simulink model "sistem_full"  (R2020b)
settings: Solver=ode45  StartTime=0.0  StopTime=10.0  MaxStep=0.01  RelTol=1e-3
undefined symbols (not defined in the file or in its folder): K_d, K_p, params, r_des
(part 2 of 2)

== matlab function sistem_full/MATLAB Function19 ==
  data: t input; coeff output; r_0 input; r_end input
function coeff  = calculation_coefficients(t, r_0, r_end)

x_0 = r_0;
x_dot_0 = 0;
x_ddot_0 = 0;

x_des = r_end;
x_dot_des = 0;
x_ddot_des = 0;

waypoints = [x_0    x_dot_0     x_ddot_0;
             x_des  x_dot_des   x_ddot_des]';
t = [0 t];

time_size = size(t);
n = 0;
%T = linspace(0, time_size(2) - 1, point(2));


border_conditions_sigm = reshape(waypoints(:, n + 1 : n + 2),1,[]);
%disp(border_conditions_sigm)

coeff = zeros(6, 1);

parameters = [1 * (t(n + 1) ^ 5), 1 * (t(n + 1) ^ 4), 1 * (t(n + 1) ^ 3), 1 * (t(n + 1) ^ 2), 1 * (t(n + 1) ^ 1), 1 * (t(n + 1) ^ 0);
              5 * (t(n + 1) ^ 4), 4 * (t(n + 1) ^ 3), 3 * (t(n + 1) ^ 2), 2 * (t(n + 1) ^ 1), 1 * (t(n + 1) ^ 0), 0 * (t(n + 1) ^ 0);
              20 * (t(n + 1) ^ 3), 12 * (t(n + 1) ^ 2), 6 * (t(n + 1) ^ 1), 2 * (t(n + 1) ^ 0), 0 * (t(n + 1) ^ 0), 0 * (t(n + 1) ^ 0);
              1 * (t(n + 2) ^ 5), 1 * (t(n + 2) ^ 4), 1 * (t(n + 2) ^ 3), 1 * (t(n + 2) ^ 2), 1 * (t(n + 2) ^ 1), 1 * (t(n + 2) ^ 0);
              5 * (t(n + 2) ^ 4), 4 * (t(n + 2) ^ 3), 3 * (t(n + 2) ^ 2), 2 * (t(n + 2) ^ 1), 1 * (t(n + 2) ^ 0), 0 * (t(n + 2) ^ 0);
              20 * (t(n + 2) ^ 3), 12 * (t(n + 2) ^ 2), 6 * (t(n + 2) ^ 1), 2 * (t(n + 2) ^ 0), 0 * (t(n + 2) ^ 0), 0 * (t(n + 2) ^ 0)];

coeff = inv(parameters) * border_conditions_sigm';

== matlab function sistem_full/MATLAB Function20 ==
  data: coeff input; pos output; clock input; vel output; acc output
function [pos, vel, acc] = trajectories_calculation(coeff, clock)

T_p = [clock^5      clock^4     clock^3     clock^2     clock   1]';
T_v = [5*clock^4    4*clock^3   3*clock^2   2*clock     1       0]';
T_a = [20*clock^3   12*clock^2  6*clock     2           0       0]';

pos = sum(coeff.*T_p);
vel = sum(coeff.*T_v);
acc = sum(coeff.*T_a);

== matlab function sistem_full/MATLAB Function21 ==
  data: t input; coeff output; r_0 input; r_end input
function coeff  = calculation_coefficients(t, r_0, r_end)

x_0 = r_0;
x_dot_0 = 14.1;
x_ddot_0 = 0;

x_des = r_end;
x_dot_des = 14.1;
x_ddot_des = 0;

waypoints = [x_0    x_dot_0     x_ddot_0;
             x_des  x_dot_des   x_ddot_des]';
t = [0 t];

time_size = size(t);
n = 0;
%T = linspace(0, time_size(2) - 1, point(2));


border_conditions_sigm = reshape(waypoints(:, n + 1 : n + 2),1,[]);
%disp(border_conditions_sigm)

coeff = zeros(6, 1);

parameters = [1 * (t(n + 1) ^ 5), 1 * (t(n + 1) ^ 4), 1 * (t(n + 1) ^ 3), 1 * (t(n + 1) ^ 2), 1 * (t(n + 1) ^ 1), 1 * (t(n + 1) ^ 0);
              5 * (t(n + 1) ^ 4), 4 * (t(n + 1) ^ 3), 3 * (t(n + 1) ^ 2), 2 * (t(n + 1) ^ 1), 1 * (t(n + 1) ^ 0), 0 * (t(n + 1) ^ 0);
              20 * (t(n + 1) ^ 3), 12 * (t(n + 1) ^ 2), 6 * (t(n + 1) ^ 1), 2 * (t(n + 1) ^ 0), 0 * (t(n + 1) ^ 0), 0 * (t(n + 1) ^ 0);
              1 * (t(n + 2) ^ 5), 1 * (t(n + 2) ^ 4), 1 * (t(n + 2) ^ 3), 1 * (t(n + 2) ^ 2), 1 * (t(n + 2) ^ 1), 1 * (t(n + 2) ^ 0);
              5 * (t(n + 2) ^ 4), 4 * (t(n + 2) ^ 3), 3 * (t(n + 2) ^ 2), 2 * (t(n + 2) ^ 1), 1 * (t(n + 2) ^ 0), 0 * (t(n + 2) ^ 0);
              20 * (t(n + 2) ^ 3), 12 * (t(n + 2) ^ 2), 6 * (t(n + 2) ^ 1), 2 * (t(n + 2) ^ 0), 0 * (t(n + 2) ^ 0), 0 * (t(n + 2) ^ 0)];

coeff = inv(parameters) * border_conditions_sigm';

== matlab function sistem_full/MATLAB Function22 ==
  data: r_des input; F_T output; Y output; fi_des output; x_ddot input; y_ddot input; z_ddot input; params input; mode input; theta_des output; psi_des output
function [F_T, Y, fi_des, theta_des, psi_des] = fcn(r_des, x_ddot, y_ddot, z_ddot, params, mode)

if mode == 0
    
    F_T = params.m * (z_ddot + params.g);
    Y = 0;

    fi_des = (1 / params.g) * (x_ddot * sin(r_des.psi) - y_ddot * cos(r_des.psi));
    theta_des = (1 / params.g) * (x_ddot * cos(r_des.psi) + y_ddot * sin(r_des.psi));
    psi_des = r_des.psi;
    
elseif mode == 1
    
    %F_T = params.m * x_ddot + params.k_x * x_dot;

    F_T = params.m * x_ddot + r_des.x_dot;
    Y = params.m * params.g;

    fi_des = r_des.fi;
    theta_des = (params.m / (params.k_x * r_des.x_dot)) * (y_ddot * sin(r_des.fi) - z_ddot * cos(r_des.fi));
    psi_des = (params.m / (params.k_x * r_des.x_dot)) * (y_ddot * cos(r_des.fi) + z_ddot * sin(r_des.fi));

    %theta_des = (params.m / F_T) * (y_ddot * sin(r_des.fi) - z_ddot * cos(r_des.fi));
    %psi_des = (params.m / F_T) * (y_ddot * cos(r_des.fi) + z_ddot * sin(r_des.fi));
    
else 
    
    F_T = params.m * (z_ddot + params.g);
    Y = 0;

    fi_des = (1 / params.g) * (x_ddot * sin(r_des.psi) - y_ddot * cos(r_des.psi));
    theta_des = (1 / params.g) * (x_ddot * cos(r_des.psi) + y_ddot * sin(r_des.psi));
    psi_des = r_des.psi;
    
end

== matlab function sistem_full/MATLAB Function23 ==
  data: alpha_1 output; alpha_2 output; alpha_3 output; alpha_4 output; F_T input; Y input; w output; M_x input; M_y input; M_z input; x_dot input; params input; alpha_L output; alpha_R output; alpha_H output; alpha_F output; mode input
function [alpha_1, alpha_2, alpha_3, alpha_4, w, alpha_L, alpha_R, alpha_H, alpha_F] = fcn(F_T, Y, M_x, M_y, M_z, x_dot, params, mode)

if mode == 0
    
    alpha_1 = (1 / (4 * params.k_Y)) * (F_T + M_x + M_y + M_z) - 7;
    alpha_2 = (1 / (4 * params.k_Y)) * (F_T + M_x - M_y - M_z);
    alpha_3 = (1 / (4 * params.k_Y)) * (F_T - M_x + M_y - M_z) - 7;
    alpha_4 = (1 / (4 * params.k_Y)) * (F_T - M_x - M_y + M_z);
    
    w = params.w_0;
    alpha_L = -7;
    alpha_R = -7;
    alpha_H = 0;
    alpha_F = 0;
    
elseif mode == 1
    
    alpha_1 = 7.5;
    alpha_2 = 7.5;
    alpha_3 = 7.5;
    alpha_4 = 7.5;

    w = (50000 * F_T + 245100) / 77;

    alpha_L = (500 * M_x + 500 * Y + 102201 * params.S_k * params.rho - 14630 * params.S_k * params.rho * x_dot) / (30 * params.S_k * params.rho * (70 * x_dot - 489));
    alpha_R = - (500 * M_x - 500 * Y - 102201 * params.S_k * params.rho + 14630 * params.S_k * params.rho * x_dot) / (30 * params.S_k * params.rho * (70 * x_dot - 489));
    alpha_H = (125 * M_y) / (3 * params.S_h * params.rho * (70 * x_dot - 489));
    alpha_F = (125 * M_z) / (3 * params.S_f * params.rho * (70 * x_dot - 489));
    
else
    
    alpha_1 = (1 / (4 * params.k_Y)) * (F_T + M_x + M_y + M_z) - 7;
    alpha_2 = (1 / (4 * params.k_Y)) * (F_T + M_x - M_y - M_z);
    alpha_3 = (1 / (4 * params.k_Y)) * (F_T - M_x + M_y - M_z) - 7;
    alpha_4 = (1 / (4 * params.k_Y)) * (F_T - M_x - M_y + M_z);
    
    w = params.w_0;
    alpha_L = -7;
    alpha_R = -7;
    alpha_H = 0;
    alpha_F = 0;
    
end

== matlab function sistem_full/MATLAB Function6 ==
  data: coeff input; pos output; clock input; vel output; acc output
function [pos, vel, acc] = trajectories_calculation(coeff, clock)

T_p = [clock^5      clock^4     clock^3     clock^2     clock   1]';
T_v = [5*clock^4    4*clock^3   3*clock^2   2*clock     1       0]';
T_a = [20*clock^3   12*clock^2  6*clock     2           0       0]';

pos = sum(coeff.*T_p);
vel = sum(coeff.*T_v);
acc = sum(coeff.*T_a);

== matlab function sistem_full/MATLAB Function ==
  data: coeff input; pos output; clock input; vel output; acc output
function [pos, vel, acc] = trajectories_calculation(coeff, clock)

T_p = [clock^5      clock^4     clock^3     clock^2     clock   1]';
T_v = [5*clock^4    4*clock^3   3*clock^2   2*clock     1       0]';
T_a = [20*clock^3   12*clock^2  6*clock     2           0       0]';

pos = sum(coeff.*T_p);
vel = sum(coeff.*T_v);
acc = sum(coeff.*T_a);

== matlab function sistem_full/MATLAB Function8 ==
  data: t input; coeff output; r_0 input; r_end input
function coeff  = calculation_coefficients(t, r_0, r_end)

x_0 = r_0;
x_dot_0 = 0;
x_ddot_0 = 0;

x_des = r_end;
x_dot_des = 0;
x_ddot_des = 0;

waypoints = [x_0    x_dot_0     x_ddot_0;
             x_des  x_dot_des   x_ddot_des]';
t = [0 t];

time_size = size(t);
n = 0;
%T = linspace(0, time_size(2) - 1, point(2));


border_conditions_sigm = reshape(waypoints(:, n + 1 : n + 2),1,[]);
%disp(border_conditions_sigm)

coeff = zeros(6, 1);

parameters = [1 * (t(n + 1) ^ 5), 1 * (t(n + 1) ^ 4), 1 * (t(n + 1) ^ 3), 1 * (t(n + 1) ^ 2), 1 * (t(n + 1) ^ 1), 1 * (t(n + 1) ^ 0);
              5 * (t(n + 1) ^ 4), 4 * (t(n + 1) ^ 3), 3 * (t(n + 1) ^ 2), 2 * (t(n + 1) ^ 1), 1 * (t(n + 1) ^ 0), 0 * (t(n + 1) ^ 0);
              20 * (t(n + 1) ^ 3), 12 * (t(n + 1) ^ 2), 6 * (t(n + 1) ^ 1), 2 * (t(n + 1) ^ 0), 0 * (t(n + 1) ^ 0), 0 * (t(n + 1) ^ 0);
              1 * (t(n + 2) ^ 5), 1 * (t(n + 2) ^ 4), 1 * (t(n + 2) ^ 3), 1 * (t(n + 2) ^ 2), 1 * (t(n + 2) ^ 1), 1 * (t(n + 2) ^ 0);
              5 * (t(n + 2) ^ 4), 4 * (t(n + 2) ^ 3), 3 * (t(n + 2) ^ 2), 2 * (t(n + 2) ^ 1), 1 * (t(n + 2) ^ 0), 0 * (t(n + 2) ^ 0);
              20 * (t(n + 2) ^ 3), 12 * (t(n + 2) ^ 2), 6 * (t(n + 2) ^ 1), 2 * (t(n + 2) ^ 0), 0 * (t(n + 2) ^ 0), 0 * (t(n + 2) ^ 0)];

coeff = inv(parameters) * border_conditions_sigm';

== matlab function sistem_full/Subsystem2/MATLAB Function6 ==
  data: x_des input; x_ddot output; x_dot_des input; x_ddot_des input; y_des input; y_dot_des input; y_ddot_des input; z_des input; z_dot_des input; z_ddot_des input; x input; x_dot input; y input; y_dot input; z input; z_dot input; K_p input; K_d input; y_ddot output; z_ddot output; mode input
function [x_ddot,y_ddot,z_ddot] = fcn(x_des, x_dot_des, x_ddot_des, y_des, y_dot_des, y_ddot_des, z_des, z_dot_des, z_ddot_des, ...
                                      x, x_dot, y, y_dot, z, z_dot, K_p, K_d, mode)

if mode == 0
    
    x_ddot = x_ddot_des + abs(K_d.ver.x) * (x_dot_des - x_dot) + abs(K_p.ver.x) * (x_des - x);
    y_ddot = y_ddot_des + abs(K_d.ver.y) * (y_dot_des - y_dot) + abs(K_p.ver.y) * (y_des - y);
    z_ddot = z_ddot_des + abs(K_d.ver.z) * (z_dot_des - z_dot) + abs(K_p.ver.z) * (z_des - z);

elseif mode == 1
    
    x_ddot = x_ddot_des + abs(K_d.hor.x) * (x_dot_des - x_dot) + abs(K_p.hor.x) * (x_des - x);
    y_ddot = y_ddot_des + abs(K_d.hor.y) * (y_dot_des - y_dot) + abs(K_p.hor.y) * (y_des - y);
    z_ddot = z_ddot_des + abs(K_d.hor.z) * (z_dot_des - z_dot) + abs(K_p.hor.z) * (z_des - z);
    
else
    
    x_ddot = x_ddot_des + abs(K_d.ver.x) * (x_dot_des - x_dot) + abs(K_p.ver.x) * (x_des - x);
    y_ddot = y_ddot_des + abs(K_d.ver.y) * (y_dot_des - y_dot) + abs(K_p.ver.y) * (y_des - y);
    z_ddot = z_ddot_des + abs(K_d.ver.z) * (z_dot_des - z_dot) + abs(K_p.ver.z) * (z_des - z);
    
end

== matlab function sistem_full/Subsystem3/MATLAB Function8 ==
  data: fi_des input; theta_des input; psi_des input; r_des input; fi input; fi_dot input; theta input; theta_dot input; psi input; psi_dot input; M_x output; K_p input; K_d input; params input; M_y output; M_z output; mode input
function [M_x, M_y, M_z] = fcn(fi_des, theta_des, psi_des, r_des, fi, fi_dot, theta, theta_dot, psi, psi_dot, K_p, K_d, params, mode)

if mode == 0

    M_x = (params.ver.J_xx / params.ver.L_x) * (r_des.fi_ddot + abs(K_d.ver.fi) * (r_des.fi_dot - fi_dot) + abs(K_p.ver.fi) * (fi_des - fi));
    M_y = (params.ver.J_yy / params.ver.L_y) * (r_des.theta_ddot + abs(K_d.ver.theta) * (r_des.theta_dot - theta_dot) + abs(K_p.ver.theta) * (theta_des - theta));
    M_z = (params.ver.J_zz / params.ver.L_z) * (r_des.psi_ddot + abs(K_d.ver.psi) * (r_des.psi_dot - psi_dot) + abs(K_p.ver.psi) * (psi_des - psi));
    
elseif mode == 1
    
    M_x = (params.hor.J_xx / params.hor.L_x) * (r_des.fi_ddot + abs(K_d.hor.fi) * (r_des.fi_dot - fi_dot) + abs(K_p.hor.fi) * (fi_des - fi));
    M_y = (params.hor.J_yy / params.hor.L_y) * (r_des.theta_ddot + abs(K_d.hor.theta) * (r_des.theta_dot - theta_dot) + abs(K_p.hor.theta) * (theta_des - theta));
    M_z = (params.hor.J_zz / params.hor.L_z) * (r_des.psi_ddot + abs(K_d.hor.psi) * (r_des.psi_dot - psi_dot) + abs(K_p.hor.psi) * (psi_des - psi));
    
else 
    
    M_x = (params.ver.J_xx / params.ver.L_x) * (r_des.fi_ddot + abs(K_d.ver.fi) * (r_des.fi_dot - fi_dot) + abs(K_p.ver.fi) * (fi_des - fi));
    M_y = (params.ver.J_yy / params.ver.L_y) * (r_des.theta_ddot + abs(K_d.ver.theta) * (r_des.theta_dot - theta_dot) + abs(K_p.ver.theta) * (theta_des - theta));
    M_z = (params.ver.J_zz / params.ver.L_z) * (r_des.psi_ddot + abs(K_d.ver.psi) * (r_des.psi_dot - psi_dot) + abs(K_p.ver.psi) * (psi_des - psi));
    
end

== matlab function sistem_full/MATLAB Function24 ==
  data: F_x input; x_ddot output; F_y input; F_z input; Y input; x_dot input; params input; y_ddot output; z_ddot output
function [x_ddot, y_ddot, z_ddot] = fcn(F_x, F_y, F_z, Y, x_dot, params)

x_ddot = (1 / params.m) * (F_x - params.k_x * x_dot);

%x_ddot = (1 / params.m) * (F_x);
y_ddot = (1 / params.m) * F_y;
z_ddot = (1 / params.m) * (F_z + Y - params.m * params.g);

== stateflow chart sistem_full/Chart2 ==
  state Vertical_flight
    mode = 0
    sigma = 0
  state Horizontal_flight
    mode = 1
    sigma = 90
  (default) -> Vertical_flight
  Horizontal_flight -> Vertical_flight : [x_dot_des < 14.1]
  Vertical_flight -> Horizontal_flight : [x_dot_des > 14.1]
  data: mode output; x_dot_des input; sigma output

== matlab function sistem_full/MATLAB Function25 ==
  data: coeff input; pos output; clock input; vel output; acc output
function [pos, vel, acc] = trajectories_calculation(coeff, clock)

T_p = [clock^5      clock^4     clock^3     clock^2     clock   1]';
T_v = [5*clock^4    4*clock^3   3*clock^2   2*clock     1       0]';
T_a = [20*clock^3   12*clock^2  6*clock     2           0       0]';

pos = sum(coeff.*T_p);
vel = sum(coeff.*T_v);
acc = sum(coeff.*T_a);

== matlab function sistem_full/MATLAB Function26 ==
  data: t input; coeff output; r_0 input; r_end input
function coeff  = calculation_coefficients(t, r_0, r_end)

x_0 = r_0;
x_dot_0 = 0;
x_ddot_0 = 0;

x_des = r_end;
x_dot_des = 0;
x_ddot_des = 0;

waypoints = [x_0    x_dot_0     x_ddot_0;
             x_des  x_dot_des   x_ddot_des]';
t = [0 t];

time_size = size(t);
n = 0;
%T = linspace(0, time_size(2) - 1, point(2));


border_conditions_sigm = reshape(waypoints(:, n + 1 : n + 2),1,[]);
%disp(border_conditions_sigm)

coeff = zeros(6, 1);

parameters = [1 * (t(n + 1) ^ 5), 1 * (t(n + 1) ^ 4), 1 * (t(n + 1) ^ 3), 1 * (t(n + 1) ^ 2), 1 * (t(n + 1) ^ 1), 1 * (t(n + 1) ^ 0);
              5 * (t(n + 1) ^ 4), 4 * (t(n + 1) ^ 3), 3 * (t(n + 1) ^ 2), 2 * (t(n + 1) ^ 1), 1 * (t(n + 1) ^ 0), 0 * (t(n + 1) ^ 0);
              20 * (t(n + 1) ^ 3), 12 * (t(n + 1) ^ 2), 6 * (t(n + 1) ^ 1), 2 * (t(n + 1) ^ 0), 0 * (t(n + 1) ^ 0), 0 * (t(n + 1) ^ 0);
              1 * (t(n + 2) ^ 5), 1 * (t(n + 2) ^ 4), 1 * (t(n + 2) ^ 3), 1 * (t(n + 2) ^ 2), 1 * (t(n + 2) ^ 1), 1 * (t(n + 2) ^ 0);
              5 * (t(n + 2) ^ 4), 4 * (t(n + 2) ^ 3), 3 * (t(n + 2) ^ 2), 2 * (t(n + 2) ^ 1), 1 * (t(n + 2) ^ 0), 0 * (t(n + 2) ^ 0);
              20 * (t(n + 2) ^ 3), 12 * (t(n + 2) ^ 2), 6 * (t(n + 2) ^ 1), 2 * (t(n + 2) ^ 0), 0 * (t(n + 2) ^ 0), 0 * (t(n + 2) ^ 0)];

coeff = inv(parameters) * border_conditions_sigm';

== stateflow chart sistem_full/Chart ==
  state Vertical_flight
    mode = 0
    sigma = 0
  state Horizontal_flight
    mode = 1
    sigma = 90
  (default) -> Vertical_flight
  Horizontal_flight -> Vertical_flight : [x_dot_des < 14.1]
  Vertical_flight -> Horizontal_flight : [x_dot_des > 14.1]
  data: mode output; x_dot_des input; sigma output

== matlab function sistem_full/MATLAB Function27 ==
  data: coeff input; pos output; clock input; vel output; acc output
function [pos, vel, acc] = trajectories_calculation(coeff, clock)

T_p = [clock^5      clock^4     clock^3     clock^2     clock   1]';
T_v = [5*clock^4    4*clock^3   3*clock^2   2*clock     1       0]';
T_a = [20*clock^3   12*clock^2  6*clock     2           0       0]';

pos = sum(coeff.*T_p);
vel = sum(coeff.*T_v);
acc = sum(coeff.*T_a);

== matlab function sistem_full/MATLAB Function28 ==
  data: t input; coeff output; r_0 input; r_end input
function coeff  = calculation_coefficients(t, r_0, r_end)

x_0 = r_0;
x_dot_0 = 14.1;
x_ddot_0 = 0;

x_des = r_end;
x_dot_des = 14.1;
x_ddot_des = 0;

waypoints = [x_0    x_dot_0     x_ddot_0;
             x_des  x_dot_des   x_ddot_des]';
t = [0 t];

time_size = size(t);
n = 0;
%T = linspace(0, time_size(2) - 1, point(2));


border_conditions_sigm = reshape(waypoints(:, n + 1 : n + 2),1,[]);
%disp(border_conditions_sigm)

coeff = zeros(6, 1);

parameters = [1 * (t(n + 1) ^ 5), 1 * (t(n + 1) ^ 4), 1 * (t(n + 1) ^ 3), 1 * (t(n + 1) ^ 2), 1 * (t(n + 1) ^ 1), 1 * (t(n + 1) ^ 0);
              5 * (t(n + 1) ^ 4), 4 * (t(n + 1) ^ 3), 3 * (t(n + 1) ^ 2), 2 * (t(n + 1) ^ 1), 1 * (t(n + 1) ^ 0), 0 * (t(n + 1) ^ 0);
              20 * (t(n + 1) ^ 3), 12 * (t(n + 1) ^ 2), 6 * (t(n + 1) ^ 1), 2 * (t(n + 1) ^ 0), 0 * (t(n + 1) ^ 0), 0 * (t(n + 1) ^ 0);
              1 * (t(n + 2) ^ 5), 1 * (t(n + 2) ^ 4), 1 * (t(n + 2) ^ 3), 1 * (t(n + 2) ^ 2), 1 * (t(n + 2) ^ 1), 1 * (t(n + 2) ^ 0);
              5 * (t(n + 2) ^ 4), 4 * (t(n + 2) ^ 3), 3 * (t(n + 2) ^ 2), 2 * (t(n + 2) ^ 1), 1 * (t(n + 2) ^ 0), 0 * (t(n + 2) ^ 0);
              20 * (t(n + 2) ^ 3), 12 * (t(n + 2) ^ 2), 6 * (t(n + 2) ^ 1), 2 * (t(n + 2) ^ 0), 0 * (t(n + 2) ^ 0), 0 * (t(n + 2) ^ 0)];

coeff = inv(parameters) * border_conditions_sigm';

== matlab function sistem_full/MATLAB Function29 ==
  data: r_des input; F_T output; Y output; fi_des output; x_ddot input; y_ddot input; z_ddot input; params input; mode input; theta_des output; psi_des output
function [F_T, Y, fi_des, theta_des, psi_des] = fcn(r_des, x_ddot, y_ddot, z_ddot, params, mode)

if mode == 0
    
    F_T = params.m * (z_ddot + params.g);
    Y = 0;

    fi_des = (1 / params.g) * (x_ddot * sin(r_des.psi) - y_ddot * cos(r_des.psi));
    theta_des = (1 / params.g) * (x_ddot * cos(r_des.psi) + y_ddot * sin(r_des.psi));
    psi_des = r_des.psi;
    
elseif mode == 1
    
    %F_T = params.m * x_ddot + params.k_x * x_dot;

    F_T = params.m * x_ddot + r_des.x_dot;
    Y = params.m * params.g;

    fi_des = r_des.fi;
    theta_des = (params.m / (params.k_x * r_des.x_dot)) * (y_ddot * sin(r_des.fi) - z_ddot * cos(r_des.fi));
    psi_des = (params.m / (params.k_x * r_des.x_dot)) * (y_ddot * cos(r_des.fi) + z_ddot * sin(r_des.fi));

    %theta_des = (params.m / F_T) * (y_ddot * sin(r_des.fi) - z_ddot * cos(r_des.fi));
    %psi_des = (params.m / F_T) * (y_ddot * cos(r_des.fi) + z_ddot * sin(r_des.fi));
    
else 
    
    F_T = params.m * (z_ddot + params.g);
    Y = 0;

    fi_des = (1 / params.g) * (x_ddot * sin(r_des.psi) - y_ddot * cos(r_des.psi));
    theta_des = (1 / params.g) * (x_ddot * cos(r_des.psi) + y_ddot * sin(r_des.psi));
    psi_des = r_des.psi;
    
end

== matlab function sistem_full/MATLAB Function30 ==
  data: alpha_1 output; alpha_2 output; alpha_3 output; alpha_4 output; F_T input; Y input; w output; M_x input; M_y input; M_z input; x_dot input; params input; alpha_L output; alpha_R output; alpha_H output; alpha_F output; mode input
function [alpha_1, alpha_2, alpha_3, alpha_4, w, alpha_L, alpha_R, alpha_H, alpha_F] = fcn(F_T, Y, M_x, M_y, M_z, x_dot, params, mode)

if mode == 0
    
    alpha_1 = (1 / (4 * params.k_Y)) * (F_T + M_x + M_y + M_z) - 7;
    alpha_2 = (1 / (4 * params.k_Y)) * (F_T + M_x - M_y - M_z);
    alpha_3 = (1 / (4 * params.k_Y)) * (F_T - M_x + M_y - M_z) - 7;
    alpha_4 = (1 / (4 * params.k_Y)) * (F_T - M_x - M_y + M_z);
    
    w = params.w_0;
    alpha_L = -7;
    alpha_R = -7;
    alpha_H = 0;
    alpha_F = 0;
    
elseif mode == 1
    
    alpha_1 = 7.5;
    alpha_2 = 7.5;
    alpha_3 = 7.5;
    alpha_4 = 7.5;

    w = (50000 * F_T + 245100) / 77;

    alpha_L = (500 * M_x + 500 * Y + 102201 * params.S_k * params.rho - 14630 * params.S_k * params.rho * x_dot) / (30 * params.S_k * params.rho * (70 * x_dot - 489));
    alpha_R = - (500 * M_x - 500 * Y - 102201 * params.S_k * params.rho + 14630 * params.S_k * params.rho * x_dot) / (30 * params.S_k * params.rho * (70 * x_dot - 489));
    alpha_H = (125 * M_y) / (3 * params.S_h * params.rho * (70 * x_dot - 489));
    alpha_F = (125 * M_z) / (3 * params.S_f * params.rho * (70 * x_dot - 489));
    
else
    
    alpha_1 = (1 / (4 * params.k_Y)) * (F_T + M_x + M_y + M_z) - 7;
    alpha_2 = (1 / (4 * params.k_Y)) * (F_T + M_x - M_y - M_z);
    alpha_3 = (1 / (4 * params.k_Y)) * (F_T - M_x + M_y - M_z) - 7;
    alpha_4 = (1 / (4 * params.k_Y)) * (F_T - M_x - M_y + M_z);
    
    w = params.w_0;
    alpha_L = -7;
    alpha_R = -7;
    alpha_H = 0;
    alpha_F = 0;
    
end

== matlab function sistem_full/MATLAB Function31 ==
  data: coeff input; pos output; clock input; vel output; acc output
function [pos, vel, acc] = trajectories_calculation(coeff, clock)

T_p = [clock^5      clock^4     clock^3     clock^2     clock   1]';
T_v = [5*clock^4    4*clock^3   3*clock^2   2*clock     1       0]';
T_a = [20*clock^3   12*clock^2  6*clock     2           0       0]';

pos = sum(coeff.*T_p);
vel = sum(coeff.*T_v);
acc = sum(coeff.*T_a);

== matlab function sistem_full/MATLAB Function32 ==
  data: t input; coeff output; r_0 input; r_end input
function coeff  = calculation_coefficients(t, r_0, r_end)

x_0 = r_0;
x_dot_0 = 0;
x_ddot_0 = 0;

x_des = r_end;
x_dot_des = 0;
x_ddot_des = 0;

waypoints = [x_0    x_dot_0     x_ddot_0;
             x_des  x_dot_des   x_ddot_des]';
t = [0 t];

time_size = size(t);
n = 0;
%T = linspace(0, time_size(2) - 1, point(2));


border_conditions_sigm = reshape(waypoints(:, n + 1 : n + 2),1,[]);
%disp(border_conditions_sigm)

coeff = zeros(6, 1);

parameters = [1 * (t(n + 1) ^ 5), 1 * (t(n + 1) ^ 4), 1 * (t(n + 1) ^ 3), 1 * (t(n + 1) ^ 2), 1 * (t(n + 1) ^ 1), 1 * (t(n + 1) ^ 0);
              5 * (t(n + 1) ^ 4), 4 * (t(n + 1) ^ 3), 3 * (t(n + 1) ^ 2), 2 * (t(n + 1) ^ 1), 1 * (t(n + 1) ^ 0), 0 * (t(n + 1) ^ 0);
              20 * (t(n + 1) ^ 3), 12 * (t(n + 1) ^ 2), 6 * (t(n + 1) ^ 1), 2 * (t(n + 1) ^ 0), 0 * (t(n + 1) ^ 0), 0 * (t(n + 1) ^ 0);
              1 * (t(n + 2) ^ 5), 1 * (t(n + 2) ^ 4), 1 * (t(n + 2) ^ 3), 1 * (t(n + 2) ^ 2), 1 * (t(n + 2) ^ 1), 1 * (t(n + 2) ^ 0);
              5 * (t(n + 2) ^ 4), 4 * (t(n + 2) ^ 3), 3 * (t(n + 2) ^ 2), 2 * (t(n + 2) ^ 1), 1 * (t(n + 2) ^ 0), 0 * (t(n + 2) ^ 0);
              20 * (t(n + 2) ^ 3), 12 * (t(n + 2) ^ 2), 6 * (t(n + 2) ^ 1), 2 * (t(n + 2) ^ 0), 0 * (t(n + 2) ^ 0), 0 * (t(n + 2) ^ 0)];

coeff = inv(parameters) * border_conditions_sigm';

== matlab function sistem_full/Subsystem4/MATLAB Function6 ==
  data: x_des input; x_ddot output; x_dot_des input; x_ddot_des input; y_des input; y_dot_des input; y_ddot_des input; z_des input; z_dot_des input; z_ddot_des input; x input; x_dot input; y input; y_dot input; z input; z_dot input; K_p input; K_d input; y_ddot output; z_ddot output; mode input
function [x_ddot,y_ddot,z_ddot] = fcn(x_des, x_dot_des, x_ddot_des, y_des, y_dot_des, y_ddot_des, z_des, z_dot_des, z_ddot_des, ...
                                      x, x_dot, y, y_dot, z, z_dot, K_p, K_d, mode)

if mode == 0
    
    x_ddot = x_ddot_des + abs(K_d.ver.x) * (x_dot_des - x_dot) + abs(K_p.ver.x) * (x_des - x);
    y_ddot = y_ddot_des + abs(K_d.ver.y) * (y_dot_des - y_dot) + abs(K_p.ver.y) * (y_des - y);
    z_ddot = z_ddot_des + abs(K_d.ver.z) * (z_dot_des - z_dot) + abs(K_p.ver.z) * (z_des - z);

elseif mode == 1
    
    x_ddot = x_ddot_des + abs(K_d.hor.x) * (x_dot_des - x_dot) + abs(K_p.hor.x) * (x_des - x);
    y_ddot = y_ddot_des + abs(K_d.hor.y) * (y_dot_des - y_dot) + abs(K_p.hor.y) * (y_des - y);
    z_ddot = z_ddot_des + abs(K_d.hor.z) * (z_dot_des - z_dot) + abs(K_p.hor.z) * (z_des - z);
    
else
    
    x_ddot = x_ddot_des + abs(K_d.ver.x) * (x_dot_des - x_dot) + abs(K_p.ver.x) * (x_des - x);
    y_ddot = y_ddot_des + abs(K_d.ver.y) * (y_dot_des - y_dot) + abs(K_p.ver.y) * (y_des - y);
    z_ddot = z_ddot_des + abs(K_d.ver.z) * (z_dot_des - z_dot) + abs(K_p.ver.z) * (z_des - z);
    
end

== matlab function sistem_full/MATLAB Function2 ==
  data: coeff input; pos output; clock input; vel output; acc output
function [pos, vel, acc] = trajectories_calculation(coeff, clock)

T_p = [clock^5      clock^4     clock^3     clock^2     clock   1]';
T_v = [5*clock^4    4*clock^3   3*clock^2   2*clock     1       0]';
T_a = [20*clock^3   12*clock^2  6*clock     2           0       0]';

pos = sum(coeff.*T_p);
vel = sum(coeff.*T_v);
acc = sum(coeff.*T_a);

== matlab function sistem_full/Subsystem5/MATLAB Function8 ==
  data: fi_des input; theta_des input; psi_des input; r_des input; fi input; fi_dot input; theta input; theta_dot input; psi input; psi_dot input; M_x output; K_p input; K_d input; params input; M_y output; M_z output; mode input
function [M_x, M_y, M_z] = fcn(fi_des, theta_des, psi_des, r_des, fi, fi_dot, theta, theta_dot, psi, psi_dot, K_p, K_d, params, mode)

if mode == 0

    M_x = (params.ver.J_xx / params.ver.L_x) * (r_des.fi_ddot + abs(K_d.ver.fi) * (r_des.fi_dot - fi_dot) + abs(K_p.ver.fi) * (fi_des - fi));
    M_y = (params.ver.J_yy / params.ver.L_y) * (r_des.theta_ddot + abs(K_d.ver.theta) * (r_des.theta_dot - theta_dot) + abs(K_p.ver.theta) * (theta_des - theta));
    M_z = (params.ver.J_zz / params.ver.L_z) * (r_des.psi_ddot + abs(K_d.ver.psi) * (r_des.psi_dot - psi_dot) + abs(K_p.ver.psi) * (psi_des - psi));
    
elseif mode == 1
    
    M_x = (params.hor.J_xx / params.hor.L_x) * (r_des.fi_ddot + abs(K_d.hor.fi) * (r_des.fi_dot - fi_dot) + abs(K_p.hor.fi) * (fi_des - fi));
    M_y = (params.hor.J_yy / params.hor.L_y) * (r_des.theta_ddot + abs(K_d.hor.theta) * (r_des.theta_dot - theta_dot) + abs(K_p.hor.theta) * (theta_des - theta));
    M_z = (params.hor.J_zz / params.hor.L_z) * (r_des.psi_ddot + abs(K_d.hor.psi) * (r_des.psi_dot - psi_dot) + abs(K_p.hor.psi) * (psi_des - psi));
    
else 
    
    M_x = (params.ver.J_xx / params.ver.L_x) * (r_des.fi_ddot + abs(K_d.ver.fi) * (r_des.fi_dot - fi_dot) + abs(K_p.ver.fi) * (fi_des - fi));
    M_y = (params.ver.J_yy / params.ver.L_y) * (r_des.theta_ddot + abs(K_d.ver.theta) * (r_des.theta_dot - theta_dot) + abs(K_p.ver.theta) * (theta_des - theta));
    M_z = (params.ver.J_zz / params.ver.L_z) * (r_des.psi_ddot + abs(K_d.ver.psi) * (r_des.psi_dot - psi_dot) + abs(K_p.ver.psi) * (psi_des - psi));
    
end

== matlab function sistem_full/MATLAB Function33 ==
  data: w_L input; F output; w_R input; alpha_1 input; alpha_2 input; alpha_3 input; alpha_4 input; params input
function F  = fcn(w_L, w_R, alpha_1, alpha_2, alpha_3, alpha_4, params)

alpha_L = alpha_1 + alpha_2;
alpha_R = alpha_3 + alpha_4;

C_Y_L = params.a_l * alpha_L^2 + params.b_l * alpha_L + params.c_l;
C_Y_R = params.a_l * alpha_R^2 + params.b_l * alpha_R + params.c_l;

F = (3/2) * params.rho * params.S_l * (C_Y_L * w_L^2 + C_Y_R * w_R^2);

== matlab function sistem_full/MATLAB Function34 ==
  data: x_dot input; y_dot input; alpha_L input; alpha_R input; params input; Y output
function Y = fcn(x_dot, y_dot, alpha_L, alpha_R, params)

C_y_L = params.a_k * alpha_L^2 + params.b_k * alpha_L + params.c_k;
C_y_R = params.a_k * alpha_R^2 + params.b_k * alpha_R + params.c_k;

Y = (1 / 2) * params.rho * (x_dot^2 + y_dot^2) * params.S_k * (C_y_L + C_y_R);

== matlab function sistem_full/MATLAB Function35 ==
  data: w_L input; w_R input; alpha_1 input; alpha_2 input; alpha_3 input; alpha_4 input; alpha_L input; alpha_R input; alpha_H input; alpha_F input; x_dot input; y_dot input; M_x output; M_y output; M_z output; params input
function [M_x, M_y, M_z] = fcn(w_L, w_R, alpha_1, alpha_2, alpha_3, alpha_4, ...
                               alpha_L, alpha_R, alpha_H, alpha_F, x_dot, y_dot, params)

C_y_L_l_x = params.a_l * (alpha_1 + alpha_2)^2 + params.b_l * (alpha_1 + alpha_2) + params.c_l;
C_y_R_l_x = params.a_l * (alpha_3 + alpha_4)^2 + params.b_l * (alpha_3 + alpha_4) + params.c_l;

C_y_L_l_yz = params.a_l * (alpha_1 - alpha_2)^2 + params.b_l * (alpha_1 - alpha_2) + params.c_l;
C_y_R_l_yz = params.a_l * (alpha_3 - alpha_4)^2 + params.b_l * (alpha_3 - alpha_4) + params.c_l;

C_y_L_k = params.a_k * alpha_L^2 + params.b_k * alpha_L + params.c_k;
C_y_R_k = params.a_k * alpha_R^2 + params.b_k * alpha_R + params.c_k;

C_y_H = params.a_h * alpha_H^3 + params.b_h * alpha_H^2 + params.c_h * alpha_H + params.d_h;
C_y_F = params.a_f * alpha_F^3 + params.b_f * alpha_F^2 + params.c_f * alpha_F + params.d_f;

M_x = ((3 / 2) * params.rho * params.S_l * (C_y_L_l_x * w_L^2 - C_y_R_l_x * w_R^2)) + ...
      ((1 / 2) * params.rho * params.S_k * (x_dot^2 + y_dot^2) * (C_y_L_k - C_y_R_k));
  
M_y = ((3 / 2) * params.rho * params.S_l * (C_y_L_l_yz * w_L^2 + C_y_R_l_yz * w_R^2)) + ...
      ((1 / 2) * C_y_H * params.rho * params.S_h * (x_dot^2 + y_dot^2));
  
M_z = ((3 / 2) * params.rho * params.S_l * (C_y_L_l_yz * w_L^2 - C_y_R_l_yz * w_R^2)) + ...
      ((1 / 2) * C_y_F * params.rho * params.S_f * (x_dot^2 + y_dot^2));

== matlab function sistem_full/MATLAB Function36 ==
  data: F input; F_x output; fi input; theta input; psi input; F_y output; F_z output; sigma input
function [F_x, F_y, F_z] = fcn(F, fi, theta, psi, sigma)

sigma = sigma * pi / 180;

F_x = F * sin(sigma) * (cos(psi) * sin(theta) + cos(theta) * sin(fi) * sin(psi)) + F * cos(sigma) * (cos(psi) * cos(theta));
F_y = F * sin(sigma) * (sin(psi) * sin(theta) - cos(psi) * cos(theta) * sin(fi)) + F * cos(sigma) * (cos(fi) * sin(psi) + cos(psi) * sin(fi) * sin(theta));
F_z = F * sin(sigma) * (cos(fi) * cos(theta)) + F * cos(sigma) * (sin(fi) * sin(psi) - cos(fi) * cos(psi) * sin(theta));

== matlab function sistem_full/MATLAB Function37 ==
  data: F_x input; x_ddot output; F_y input; F_z input; Y input; x_dot input; y_dot input; z_dot input; params input; y_ddot output; z_ddot output
function [x_ddot, y_ddot, z_ddot] = fcn(F_x, F_y, F_z, Y, x_dot, y_dot, z_dot, params)

x_ddot = (1 / params.m) * (F_x - params.k_x * x_dot);
y_ddot = (1 / params.m) * (F_y - params.k_y * y_dot);
z_ddot = (1 / params.m) * (F_z + Y - params.k_z * z_dot - params.m * params.g);

== matlab function sistem_full/MATLAB Function3 ==
  data: t input; coeff output; r_0 input; r_end input
function coeff  = calculation_coefficients(t, r_0, r_end)

x_0 = r_0;
x_dot_0 = 0;
x_ddot_0 = 0;

x_des = r_end;
x_dot_des = 0;
x_ddot_des = 0;

waypoints = [x_0    x_dot_0     x_ddot_0;
             x_des  x_dot_des   x_ddot_des]';
t = [0 t];

time_size = size(t);
n = 0;
%T = linspace(0, time_size(2) - 1, point(2));


border_conditions_sigm = reshape(waypoints(:, n + 1 : n + 2),1,[]);
%disp(border_conditions_sigm)

coeff = zeros(6, 1);

parameters = [1 * (t(n + 1) ^ 5), 1 * (t(n + 1) ^ 4), 1 * (t(n + 1) ^ 3), 1 * (t(n + 1) ^ 2), 1 * (t(n + 1) ^ 1), 1 * (t(n + 1) ^ 0);
              5 * (t(n + 1) ^ 4), 4 * (t(n + 1) ^ 3), 3 * (t(n + 1) ^ 2), 2 * (t(n + 1) ^ 1), 1 * (t(n + 1) ^ 0), 0 * (t(n + 1) ^ 0);
              20 * (t(n + 1) ^ 3), 12 * (t(n + 1) ^ 2), 6 * (t(n + 1) ^ 1), 2 * (t(n + 1) ^ 0), 0 * (t(n + 1) ^ 0), 0 * (t(n + 1) ^ 0);
              1 * (t(n + 2) ^ 5), 1 * (t(n + 2) ^ 4), 1 * (t(n + 2) ^ 3), 1 * (t(n + 2) ^ 2), 1 * (t(n + 2) ^ 1), 1 * (t(n + 2) ^ 0);
              5 * (t(n + 2) ^ 4), 4 * (t(n + 2) ^ 3), 3 * (t(n + 2) ^ 2), 2 * (t(n + 2) ^ 1), 1 * (t(n + 2) ^ 0), 0 * (t(n + 2) ^ 0);
              20 * (t(n + 2) ^ 3), 12 * (t(n + 2) ^ 2), 6 * (t(n + 2) ^ 1), 2 * (t(n + 2) ^ 0), 0 * (t(n + 2) ^ 0), 0 * (t(n + 2) ^ 0)];

coeff = inv(parameters) * border_conditions_sigm';

== matlab function sistem_full/MATLAB Function4 ==
  data: coeff input; pos output; clock input; vel output; acc output
function [pos, vel, acc] = trajectories_calculation(coeff, clock)

T_p = [clock^5      clock^4     clock^3     clock^2     clock   1]';
T_v = [5*clock^4    4*clock^3   3*clock^2   2*clock     1       0]';
T_a = [20*clock^3   12*clock^2  6*clock     2           0       0]';

pos = sum(coeff.*T_p);
vel = sum(coeff.*T_v);
acc = sum(coeff.*T_a);

== matlab function sistem_full/Subsystem/MATLAB Function6 ==
  data: x_des input; x_ddot output; x_dot_des input; x_ddot_des input; y_des input; y_dot_des input; y_ddot_des input; z_des input; z_dot_des input; z_ddot_des input; x input; x_dot input; y input; y_dot input; z input; z_dot input; K_p input; K_d input; y_ddot output; z_ddot output; mode input
function [x_ddot,y_ddot,z_ddot] = fcn(x_des, x_dot_des, x_ddot_des, y_des, y_dot_des, y_ddot_des, z_des, z_dot_des, z_ddot_des, ...
                                      x, x_dot, y, y_dot, z, z_dot, K_p, K_d, mode)

if mode == 0
    
    x_ddot = x_ddot_des + abs(K_d.ver.x) * (x_dot_des - x_dot) + abs(K_p.ver.x) * (x_des - x);
    y_ddot = y_ddot_des + abs(K_d.ver.y) * (y_dot_des - y_dot) + abs(K_p.ver.y) * (y_des - y);
    z_ddot = z_ddot_des + abs(K_d.ver.z) * (z_dot_des - z_dot) + abs(K_p.ver.z) * (z_des - z);

elseif mode == 1
    
    x_ddot = x_ddot_des + abs(K_d.hor.x) * (x_dot_des - x_dot) + abs(K_p.hor.x) * (x_des - x);
    y_ddot = y_ddot_des + abs(K_d.hor.y) * (y_dot_des - y_dot) + abs(K_p.hor.y) * (y_des - y);
    z_ddot = z_ddot_des + abs(K_d.hor.z) * (z_dot_des - z_dot) + abs(K_p.hor.z) * (z_des - z);
    
else
    
    x_ddot = x_ddot_des + abs(K_d.ver.x) * (x_dot_des - x_dot) + abs(K_p.ver.x) * (x_des - x);
    y_ddot = y_ddot_des + abs(K_d.ver.y) * (y_dot_des - y_dot) + abs(K_p.ver.y) * (y_des - y);
    z_ddot = z_ddot_des + abs(K_d.ver.z) * (z_dot_des - z_dot) + abs(K_p.ver.z) * (z_des - z);
    
end
